simulink model "preg3_simu"  (R2021a)
settings: Solver=VariableStepAuto  StartTime=0.0  StopTime=10.0  RelTol=1e-3
values from neighbouring files (symbols this model uses):
  a = 2    [preg3.m]
  k2 = 17/60    (= 0.283333333333)    [preg3.m]
settings Model: Creator=pierr  LastModifiedBy=pierr

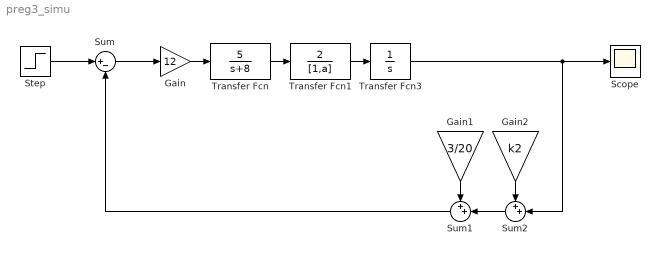
== system preg3_simu ==
  Gain : Gain  Gain=12
  Gain1 : Gain  Gain=3/20
  Gain2 : Gain  Gain=k2
  Scope : Scope
  Step : Step  SampleTime=0
  Sum : Sum  Inputs=|+-
  Sum1 : Sum  Inputs=++|
  Sum2 : Sum  Inputs=++|
  Transfer Fcn : TransferFcn  Numerator=[5]  Denominator=[1 8]
  Transfer Fcn1 : TransferFcn  Numerator=[2]  Denominator=[1,a]
  Transfer Fcn3 : TransferFcn  Denominator=[1 0]
  wires:
  Sum/1 -> Gain/1
  Gain/1 -> Transfer Fcn/1
  Transfer Fcn/1 -> Transfer Fcn1/1
  Transfer Fcn1/1 -> Transfer Fcn3/1
  Gain1/1 -> Sum1/1
  Gain2/1 -> Sum2/1
  Sum2/1 -> Sum1/2
  Sum1/1 -> Sum/2
  Transfer Fcn3/1 -> Scope/1, Sum2/2
  Step/1 -> Sum/1
